simulink model "Aula_Intro"  (R2018a)
settings: Solver=ode23  StartTime=0.0  StopTime=10.0  RelTol=1e-3
undefined symbols (not defined in the file): c, k, m
settings Model: Creator=mfant  LastModifiedBy=mfant

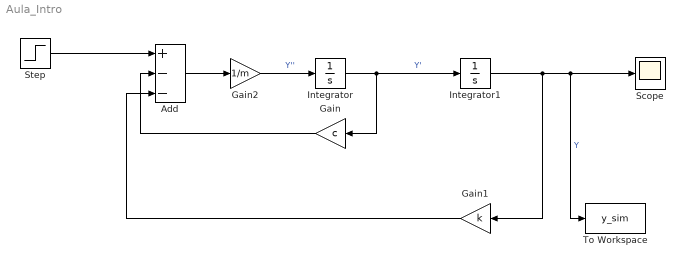
== system Aula_Intro ==
  Add : Sum  Inputs=+--
  Gain : Gain  Gain=c
  Gain1 : Gain  Gain=k
  Gain2 : Gain  Gain=1/m
  Integrator : Integrator
  Integrator1 : Integrator
  Scope : Scope
  Step : Step  Time=0  SampleTime=0
  To Workspace : ToWorkspace  VariableName=y_sim  SaveFormat=Timeseries  SampleTime=-1
  wires:
  Add/1 -> Gain2/1
  Integrator/1 -> Gain/1, Integrator1/1  "Y'"
  Integrator1/1 -> Gain1/1, To Workspace/1, Scope/1  "Y"
  Gain/1 -> Add/2
  Gain1/1 -> Add/3
  Step/1 -> Add/1
  Gain2/1 -> Integrator/1  "Y''"
